simulink model "RobotArm"  (R2024b)
settings: Solver=FixedStepDiscrete  StartTime=0.0  StopTime=inf  RelTol=1e-3
libraries: arduinolib x12
settings Model: ExtModeTrigDuration=2  Creator=Alize  LastModifiedBy=Alize
settings SolverCC: AutoInsertRateTranBlk=on
settings OptimizationCC: EnhancedBackFolding=on  PassReuseOutputArgsAs=Individual arguments  ZeroExternalMemoryAtStartup=off  ZeroInternalMemoryAtStartup=off  MaxStackSize=64  OptimizeBlockOrder=speed  DifferentSizesBufferReuse=on  OptimizationCustomize=off  EfficientTunableParamExpr=on
settings DebuggingCC: ParameterTunabilityLossMsg=error
settings HardwareCC: ProdBitPerInt=16  ProdBitPerPointer=16  ProdBitPerSizeT=16  ProdBitPerPtrDiffT=16  ProdLargestAtomicFloat=None  ProdWordSize=8  ProdHWDeviceType=Atmel->AVR
settings SFSimCC: MATLABDynamicMemAlloc=off
settings RTWCC: Description=Embedded Coder  SystemTargetFile=ert.tlc  HardwareBoard=Arduino Uno  TemplateMakefile=ert_default_tmf  Toolchain=Arduino AVR  BuildConfiguration=Faster Runs
settings CodeAppCC: ForceParamTrailComments=on  IgnoreCustomStorageClasses=off  OperatorAnnotations=on  SimulinkDataObjDesc=on  SFDataObjDesc=on  InsertBlockDesc=on
settings ERTTargetCC: SupportContinuousTime=on  SupportVariableSizeSignals=on  ExtModeTransport=3  ExtModeStaticAlloc=on  ExtModeAutomaticAllocSize=off  ExtModeStaticAllocSize=250  ExtModeMexFile=ext_xcp  ExtModeIntrfLevel=Level2 - Open  InlinedParameterPlacement=Hierarchical

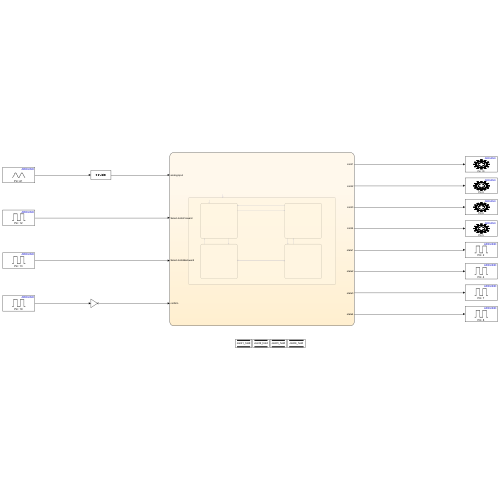
[thumbnail: Simulink's stored preview of the top-level diagram]
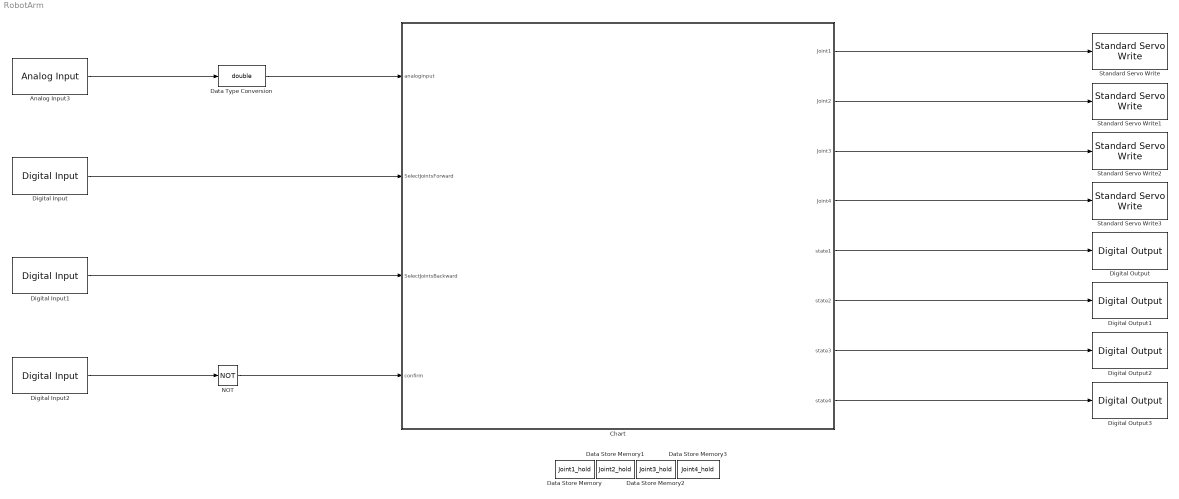
== system RobotArm ==
  Analog Input3 : arduinolib/Analog Input  pinNumber=1  ReadResultsOnly=off  ConversionTriggerSource=Software  ExternalTriggerType=uint32( 0 )  OutputDataType=uint16  EnableConversionCompleteNotify=off  EnableOuputStatus=off  SampleTime=-1  blockPlatform=arduino
  Chart : Stateflow chart  TreatAsAtomicUnit=on
  Data Store Memory : DataStoreMemory  DataStoreName=Joint1_hold  WriteAfterWriteMsg=warning  InitialValue=90  ShowAdditionalParam=off  OutDataTypeStr=double  Dimensions=1
  Data Store Memory1 : DataStoreMemory  DataStoreName=Joint2_hold  WriteAfterWriteMsg=warning  InitialValue=90  ShowAdditionalParam=off  OutDataTypeStr=double  Dimensions=1
  Data Store Memory2 : DataStoreMemory  DataStoreName=Joint3_hold  WriteAfterWriteMsg=warning  InitialValue=90  ShowAdditionalParam=off  OutDataTypeStr=double  Dimensions=1
  Data Store Memory3 : DataStoreMemory  DataStoreName=Joint4_hold  WriteAfterWriteMsg=warning  InitialValue=90  ShowAdditionalParam=off  OutDataTypeStr=double  Dimensions=1
  Data Type Conversion : DataTypeConversion  OutDataTypeStr=double  SaturateOnIntegerOverflow=off  RndMeth=Floor
  Digital Input : arduinolib/Digital Input  pinNumber=12  mode=Input Pullup  Direction=input  SampleTime=0.1  blockPlatform=arduino
  Digital Input1 : arduinolib/Digital Input  pinNumber=13  mode=Input Pullup  Direction=input  SampleTime=0.1  blockPlatform=arduino
  Digital Input2 : arduinolib/Digital Input  pinNumber=19  mode=Input Pullup  Direction=input  SampleTime=0.1  blockPlatform=arduino
  Digital Output : arduinolib/Digital Output  pinNumber=2  Direction=output  blockPlatform=arduino
  Digital Output1 : arduinolib/Digital Output  pinNumber=4  Direction=output  blockPlatform=arduino
  Digital Output2 : arduinolib/Digital Output  pinNumber=7  Direction=output  blockPlatform=arduino
  Digital Output3 : arduinolib/Digital Output  pinNumber=8  Direction=output  blockPlatform=arduino
  NOT : Logic  Operator=NOT  IconShape=distinctive  AllPortsSameDT=off  OutDataTypeStr=boolean
  Standard Servo Write : arduinolib/Standard Servo Write  pinNumber=10  ServoIndex=0  blockPlatform=ARDUINO
  Standard Servo Write1 : arduinolib/Standard Servo Write  pinNumber=9  ServoIndex=1  blockPlatform=ARDUINO
  Standard Servo Write2 : arduinolib/Standard Servo Write  pinNumber=6  ServoIndex=2  blockPlatform=ARDUINO
  Standard Servo Write3 : arduinolib/Standard Servo Write  pinNumber=5  ServoIndex=3  blockPlatform=ARDUINO
  wires:
  Analog Input3/1 -> Data Type Conversion/1
  Data Type Conversion/1 -> Chart/1(analoginput)
  Chart/5(state1) -> Digital Output/1
  Chart/6(state2) -> Digital Output1/1
  Chart/7(state3) -> Digital Output2/1
  Chart/8(state4) -> Digital Output3/1
  Digital Input/1 -> Chart/2(SelectJointsForward)
  Digital Input1/1 -> Chart/3(SelectJointsBackward)
  Digital Input2/1 -> NOT/1
  NOT/1 -> Chart/4(confirm)
  Chart/1(Joint1) -> Standard Servo Write/1
  Chart/2(Joint2) -> Standard Servo Write1/1
  Chart/3(Joint3) -> Standard Servo Write2/1
  Chart/4(Joint4) -> Standard Servo Write3/1

== stateflow chart RobotArm/Chart ==
  state Robot
    entry:
    Joint1_hold = 90;
    Joint2_hold = 90;
    Joint3_hold = 90;
    Joint4_hold = 90;
    state J1
      entry:
      state1 = 1; state2 = 0; state3 = 0; state4 = 0;
      ready = true;
      adjust_enabled = false;
      during:
      if ready && (confirm == 1)
      adjust_enabled = true;
      ready = false;
      end
      if adjust_enabled
      Joint1_hold = 90 + ((double(analoginput)/1023.0 - 0.5) * 180);
      end
      Joint1 = Joint1_hold;
      Joint2 = Joint2_hold;
      Joint3 = Joint3_hold;
      Joint4 = Joint4_hold;
    state J4
      entry:
      state4 = 1; state2 = 0; state3 = 0; state1 = 0;
      ready = true;
      adjust_enabled = false;
      during:
      if ready && (confirm == 1)
      adjust_enabled = true;
      ready = false;
      end
      if adjust_enabled
      Joint4_hold = 90 + ((double(analoginput)/1023.0 - 0.5) * 180);
      end
      Joint1 = Joint1_hold;
      Joint2 = Joint2_hold;
      Joint3 = Joint3_hold;
      Joint4 = Joint4_hold;
    state J2
      entry:
      state1 = 0; state2 = 1; state3 = 0; state4 = 0;
      ready = true;
      adjust_enabled = false;
      during:
      if ready && (confirm == 1)
      adjust_enabled = true;
      ready = false;
      end
      if adjust_enabled
      Joint2_hold = 90 + ((double(analoginput)/1023.0 - 0.5) * 180);
      end
      Joint1 = Joint1_hold;
      Joint2 = Joint2_hold;
      Joint3 = Joint3_hold;
      Joint4 = Joint4_hold;
    state J3
      entry:
      state1 = 0; state2 = 0; state3 = 1; state4 = 0;
      ready = true;
      adjust_enabled = false;
      during:
      if ready && (confirm == 1)
      adjust_enabled = true;
      ready = false;
      end
      if adjust_enabled
      Joint3_hold = 90 + ((double(analoginput)/1023.0 - 0.5) * 180);
      end
      Joint1 = Joint1_hold;
      Joint2 = Joint2_hold;
      Joint3 = Joint3_hold;
      Joint4 = Joint4_hold;
    (default) -> J1
    J4 -> J1 [order 2] : [duration(SelectJointsForward == 0) >= 3]
    J1 -> J4 [order 2] : [duration(SelectJointsBackward == 0) >= 3]
    J2 -> J1 [order 2] : [duration(SelectJointsBackward == 0) >= 3]
    J1 -> J2 [order 1] : [duration(SelectJointsForward == 0) >= 3]
    J4 -> J3 [order 1] : [duration(SelectJointsBackward == 0) >= 3]
    J3 -> J4 [order 1] : [duration(SelectJointsForward == 0) >= 3]
    J3 -> J2 [order 2] : [duration(SelectJointsBackward == 0) >= 3]
    J2 -> J3 [order 1] : [duration(SelectJointsForward == 0) >= 3]
  (default) -> Robot
  data: analoginput input; SelectJointsForward input boolean; SelectJointsBackward input boolean; Joint1 output double; Joint2 output double; Joint3 output double; Joint4 output double; state1 output; state2 output; state3 output; state4 output; Joint1_hold data_store_memory; Joint3_hold data_store_memory; Joint2_hold data_store_memory; Joint4_hold data_store_memory; confirm input boolean; ready local boolean; adjust_enabled local
